simulink model "L2_T2_current_loop"  (R2026a)
settings: Solver=ode23tb  StartTime=0  StopTime=0.008  MaxStep=2e-05
settings Model: Creator=m  LastModifiedBy=m

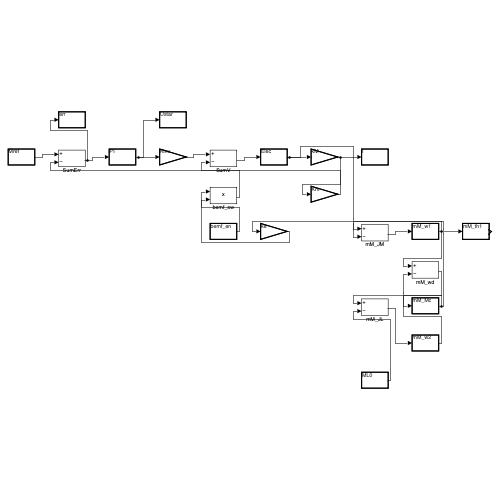
[thumbnail: Simulink's stored preview of the top-level diagram]
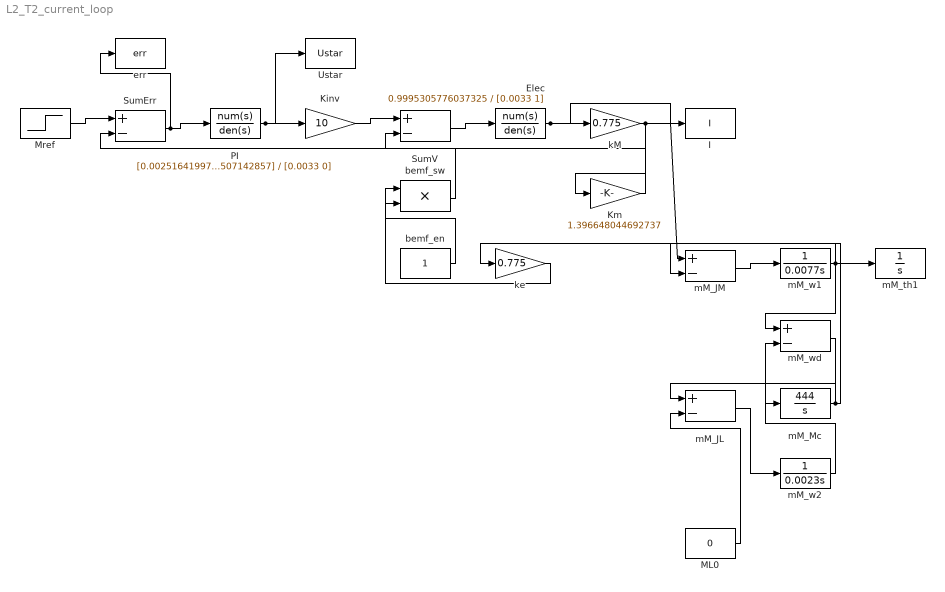
== system L2_T2_current_loop ==
  Elec : TransferFcn  Numerator=0.9995305776037325  Denominator=[0.0033 1]
  I : ToWorkspace  VariableName=I  SaveFormat=Structure With Time  SampleTime=-1
  Kinv : Gain  Gain=10
  Km : Gain  Gain=1.396648044692737
  ML0 : Constant  Value=0
  Mref : Step  Time=0  FinalValue=10  SampleTime=0
  PI : TransferFcn  Numerator=[0.002516419973571428 0.762551507142857]  Denominator=[0.0033 0]
  SumErr : Sum  Inputs=+-
  SumV : Sum  Inputs=+-
  Ustar : ToWorkspace  VariableName=Ustar  SaveFormat=Structure With Time  SampleTime=-1
  bemf_en : Constant
  bemf_sw : Product
  err : ToWorkspace  VariableName=err  SaveFormat=Structure With Time  SampleTime=-1
  kM : Gain  Gain=0.775
  ke : Gain  Gain=0.775
  mM_JL : Sum  Inputs=+-
  mM_JM : Sum  Inputs=+-
  mM_Mc : TransferFcn  Numerator=444  Denominator=[1 0]
  mM_th1 : Integrator
  mM_w1 : TransferFcn  Numerator=1  Denominator=[0.0077 0]
  mM_w2 : TransferFcn  Numerator=1  Denominator=[0.0023 0]
  mM_wd : Sum  Inputs=+-
  wires:
  mM_JM/1 -> mM_w1/1
  mM_w1/1 -> mM_wd/1, mM_th1/1, ke/1
  mM_w2/1 -> mM_wd/2
  mM_wd/1 -> mM_Mc/1
  mM_Mc/1 -> mM_JM/2, mM_JL/1
  mM_JL/1 -> mM_w2/1
  Mref/1 -> SumErr/1
  PI/1 -> Kinv/1, Ustar/1
  Kinv/1 -> SumV/1
  SumV/1 -> Elec/1
  Elec/1 -> kM/1, I/1
  kM/1 -> mM_JM/1, Km/1
  ML0/1 -> mM_JL/2
  ke/1 -> bemf_sw/1
  bemf_en/1 -> bemf_sw/2
  bemf_sw/1 -> SumV/2
  Km/1 -> SumErr/2
  SumErr/1 -> PI/1, err/1
